simulink model "ring_filter"  (R2016b)
settings: Solver=ode15s  StartTime=0.0  StopTime=6e-8  FixedStep=200e-15  MaxStep=50e-15  MinStep=1e-15  RelTol=1e-3  EnableMultiTasking=on
undefined symbols (not defined in the file): L, P_laser, t_drop, t_in, Temp
libraries: SiPhotonics x3, simulink x1
settings Model: Creator=lins08  LastModifiedBy=lins08
settings SolverCC: InitialStep=50e-15  SolverResetMethod=Robust
settings DataIOCC: LimitDataPoints=on  SaveFormat=Array
settings OptimizationCC: LifeSpan=inf
settings DebuggingCC: SFUnexpectedBacktrackingDiag=warning  SFNoUnconditionalDefaultTransitionDiag=warning  SFExecutionAtInitializationDiag=none
settings HardwareCC: ProdBitPerPointer=32  ProdBitPerSizeT=32  ProdBitPerPtrDiffT=32  ProdLargestAtomicFloat=None  ProdIntDivRoundTo=Undefined  ProdEndianess=Unspecified  ProdWordSize=32  ProdHWDeviceType=32-bit Generic
settings ModelReferenceCC: PropagateSignalLabelsOutOfModel=off
settings GRTTargetCC: TargetLangStandard=C89/C90 (ANSI)  GeneratePreprocessorConditionals=Disable all
settings ConfigComp: CovMetricSettings=dw  CovHtmlReporting=on  CovSaveCumulativeToWorkspaceVar=on  CovSaveSingleToWorkspaceVar=on  CovExternalEMLEnable=off

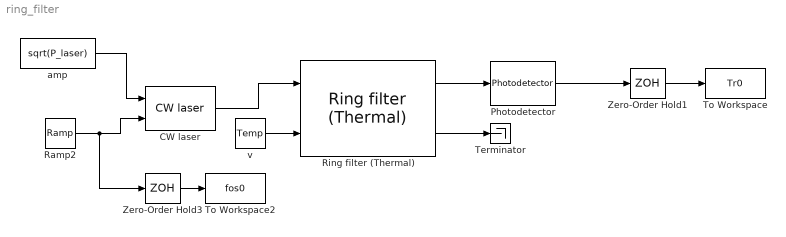
== system ring_filter ==
  CW laser : SiPhotonics/CW laser
  Photodetector : SiPhotonics/Photodetector  R=1  fbw=1e11
  Ramp2 : simulink/Sources/Ramp  slope=1e18  start=0  X0=0
  Ring filter (Thermal) : SiPhotonics/Ring filter (Thermal)  L=L  t_in=t_in  k_in=sqrt(1-t_in^2)*1i  t_drop=t_drop  k_drop=sqrt(1-t_drop^2)*1i  fref=fref  n0=n0  ng=ng  f0=f0  nt=nt  T0=T0  gamma_t=gamma_t
  Terminator : Terminator
  To Workspace : ToWorkspace  VariableName=Tr0  SaveFormat=Timeseries  SampleTime=-1
  To Workspace2 : ToWorkspace  VariableName=fos0  SaveFormat=Timeseries  SampleTime=-1
  Zero-Order Hold1 : ZeroOrderHold  SampleTime=1e-12
  Zero-Order Hold3 : ZeroOrderHold  SampleTime=1e-12
  amp : Constant  Value=sqrt(P_laser)
  v : Constant  Value=Temp
  wires:
  CW laser/1 -> Ring filter (Thermal)/1
  Ramp2/1 -> Zero-Order Hold3/1, CW laser/2
  amp/1 -> CW laser/1
  Ring filter (Thermal)/2 -> Terminator/1
  Ring filter (Thermal)/1 -> Photodetector/1
  Photodetector/1 -> Zero-Order Hold1/1
  Zero-Order Hold1/1 -> To Workspace/1
  Zero-Order Hold3/1 -> To Workspace2/1
  v/1 -> Ring filter (Thermal)/2
